simulink model "CiMappedEngine"  (R2021a)
settings: Solver=VariableStepAuto  StartTime=0.0  StopTime=inf  RelTol=1e-3  EnableMultiTasking=on
model workspace (MAT data in the model file):
  AccPwrbp = [0 0]
  AccSpdbp = [300 750]
  Cps = 2
  NCyl = 4
  Pstd = 101325
  Rair = 287.05
  Sinj = 6.45161290323
  TimeCnstECP = 0.125
  TimeCnstEGR = 0.125
  TimeCnstETC = 0.085
  TimeCnstICP = 0.125
  TimeCnstIVL = 0.125
  TimeCnstSWVA = 0.125
  TimeCnstVCR = 0.125
  TimeCnstVGT = 0.15
  TimeCnstVIRL = 0.125
  TimeCnstWGA = 0.15
  Tstd = 293.15
  Vd = 0.0015
  f_air = [0 0 0 0 0 0 0 0 0 0 0 0 ... (320 elements, 20x16)]
  f_air_3d = [0 0 0 0 0 0 0 0 0 0 0 0 ... (960 elements, 20x16x3)]
  f_co = [0 0 0 0 0 0 0 0 0 0 0 0 ... (320 elements, 20x16)]
  f_co2 = [0 0 0 0 0 0 0 0 0 0 0 0 ... (320 elements, 20x16)]
  f_co2_3d = [0 0 0 0 0 0 0 0 0 0 0 0 ... (960 elements, 20x16x3)]
  f_co_3d = [0 0 0 0 0 0 0 0 0 0 0 0 ... (960 elements, 20x16x3)]
  f_eff = [0 0 0 0 0 0 0 0 0 0 0 0 ... (320 elements, 20x16)]
  f_eff_3d = [0 0 0 0 0 0 0 0 0 0 0 0 ... (960 elements, 20x16x3)]
  f_fuel = [0 0 0 0 0 0 0 0 0 0 0 0 ... (320 elements, 20x16)]
  f_fuel_3d = [0 0 0 0 0 0 0 0 0 0 0 0 ... (960 elements, 20x16x3)]
  f_hc = [0 0 0 0 0 0 0 0 0 0 0 0 ... (320 elements, 20x16)]
  f_hc_3d = [0 0 0 0 0 0 0 0 0 0 0 0 ... (960 elements, 20x16x3)]
  f_nox = [0 0 0 0 0 0 0 0 0 0 0 0 ... (320 elements, 20x16)]
  f_nox_3d = [0 0 0 0 0 0 0 0 0 0 0 0 ... (960 elements, 20x16x3)]
  f_pm = [0 0 0 0 0 0 0 0 0 0 0 0 ... (320 elements, 20x16)]
  f_pm_3d = [0 0 0 0 0 0 0 0 0 0 0 0 ... (960 elements, 20x16x3)]
  f_tbrake = [0 15 15 15 15 15 15 15 15 15 15 15 ... (320 elements, 20x16)]
  f_tbrake_3d = [0 4.32139921766 20.7572447114 35.9627269415 49.855265726 62.5657141177 74.4770044016 86.1003984024 97.7334079818 109.479762957 121.326441846 133.101497884 ... (960 elements, 20x16x3)]
  f_tbrake_f_bpt = [0 2.63157894737 5.26315789474 7.89473684211 10.5263157895 13.1578947368 15.7894736842 18.4210526316 21.0526315789 23.6842105263 26.3157894737 28.9473684211 ... (20 elements, 1x20)]
  f_tbrake_n_bpt = [0 1000 1285.71428571 1571.42857143 1857.14285714 2142.85714286 2428.57142857 2714.28571429 3000 3285.71428571 3571.42857143 3857.14285714 ... (16 elements, 1x16)]
  f_tbrake_t_bpt = [0 4.017 21.26 37.37 52.22 65.88 78.77 91.44 104.2 116.8 129.3 141.4 ... (20 elements, 1x20)]
  f_texh = [530.615953519 585.141308787 621.791548793 637.74644696 668.027558986 729.99378178 762.870339995 814.420601609 844.420048857 859.04703204 894.926983859 943.665474082 ... (320 elements, 20x16)]
  f_texh_3d = [358.711368346 410.521929896 465.556483184 518.480956339 566.158596806 618.256764358 675.886138918 720.044246232 742.940029896 751.128194054 760.390444558 779.777710435 ... (960 elements, 20x16x3)]
libraries: autolibpowerinfoutils x1, autolibsharedmappedengines x1
(part 2 of 2)

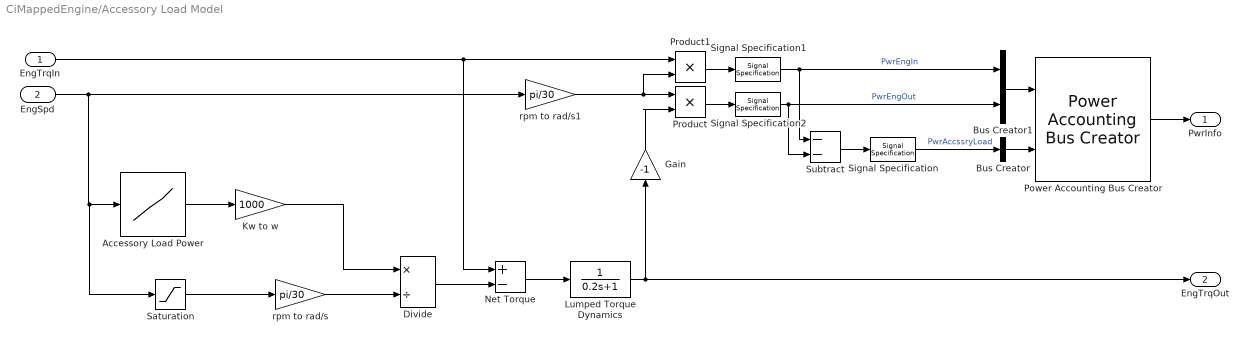
== system CiMappedEngine/Accessory Load Model ==
  EngTrqIn : Inport
  EngSpd : Inport  Port=2
  Accessory Load Power : Lookup_n-D  NumberOfTableDimensions=1  LookupTableObject=''  BreakpointsForDimension1=AccSpdbp  Table=AccPwrbp  ExtrapMethod=Clip  InternalRulePriority=Speed  RndMeth=Simplest  InputSameDT=on
  Bus Creator : BusCreator  Inputs=1
  Bus Creator1 : BusCreator  Inputs=2
  Divide : Product  Inputs=*/
  Gain : Gain  Gain=-1
  Kw to w : Gain  Gain=1000
  Lumped Torque Dynamics : TransferFcn  Denominator=[0.2 1]
  Net Torque : Sum  Inputs=+-
  Power Accounting Bus Creator : autolibpowerinfoutils/Power Accounting Bus Creator  AssctBlkSelPopup=Parent  RefBlkName='libraryname/blkname'  PwrTrnsfrdCheckBox=on  PwrNotTrnsfrdCheckBox=on  PwrStoredCheckBox=off  aMode=aMode
      settings: SourceProductBaseCode=PW,DR,MT,UV,VE
  Product : Product
  Product1 : Product
  Saturation : Saturate  UpperLimit=Inf  LowerLimit=300
  Signal Specification : SignalSpecification  Unit=W
  Signal Specification1 : SignalSpecification  Unit=W
  Signal Specification2 : SignalSpecification  Unit=W
  Subtract : Sum  Inputs=--
  rpm to rad/s : Gain  Gain=pi/30
  rpm to rad/s1 : Gain  Gain=pi/30
  PwrInfo : Outport  VectorParamsAs1DForOutWhenUnconnected=off
  EngTrqOut : Outport  Port=2  Unit=N*m  VectorParamsAs1DForOutWhenUnconnected=off
  wires:
  Divide/1 -> Net Torque/2
  Accessory Load Power/1 -> Kw to w/1
  EngSpd/1 -> Saturation/1, Accessory Load Power/1, rpm to rad/s1/1
  Saturation/1 -> rpm to rad/s/1
  rpm to rad/s/1 -> Divide/2
  Lumped Torque Dynamics/1 -> EngTrqOut/1, Gain/1
  Net Torque/1 -> Lumped Torque Dynamics/1
  Bus Creator/1 -> Power Accounting Bus Creator/2
  Kw to w/1 -> Divide/1
  Bus Creator1/1 -> Power Accounting Bus Creator/1
  EngTrqIn/1 -> Product1/1, Net Torque/1
  Subtract/1 -> Signal Specification/1
  Signal Specification/1 -> Bus Creator/1  "PwrAccssryLoad"
  Power Accounting Bus Creator/1 -> PwrInfo/1
  Product/1 -> Signal Specification2/1
  Product1/1 -> Signal Specification1/1
  rpm to rad/s1/1 -> Product1/2, Product/1
  Signal Specification1/1 -> Subtract/1, Bus Creator1/1  "PwrEngIn"
  Signal Specification2/1 -> Subtract/2, Bus Creator1/2  "PwrEngOut"
  Gain/1 -> Product/2

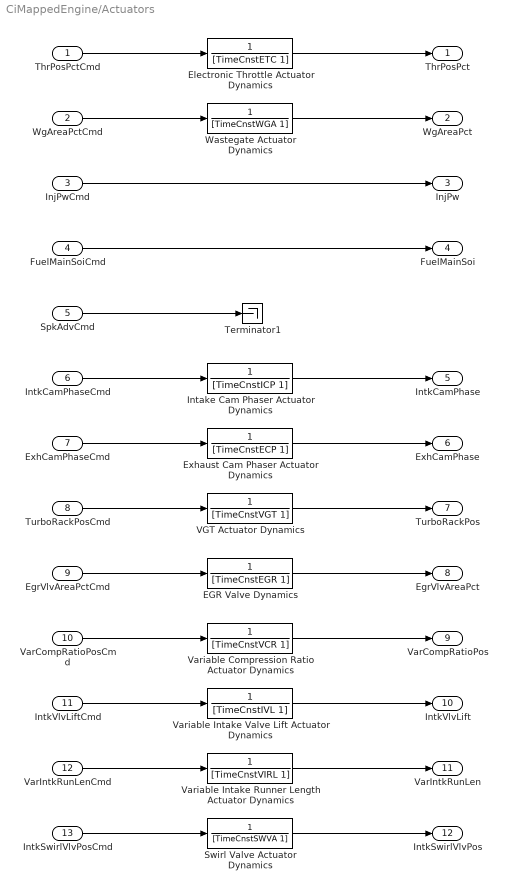
== system CiMappedEngine/Actuators ==
  ThrPosPctCmd : Inport  Unit=%
  WgAreaPctCmd : Inport  Port=2  Unit=%
  InjPwCmd : Inport  Port=3  Unit=ms
  FuelMainSoiCmd : Inport  Port=4  Unit=deg
  SpkAdvCmd : Inport  Port=5  Unit=deg
  IntkCamPhaseCmd : Inport  Port=6  Unit=deg
  ExhCamPhaseCmd : Inport  Port=7  Unit=deg
  TurboRackPosCmd : Inport  Port=8  Unit=1
  EgrVlvAreaPctCmd : Inport  Port=9  Unit=%
  VarCompRatioPosCmd : Inport  Port=10
  IntkVlvLiftCmd : Inport  Port=11
  VarIntkRunLenCmd : Inport  Port=12
  IntkSwirlVlvPosCmd : Inport  Port=13
  EGR Valve Dynamics : TransferFcn  Denominator=[TimeCnstEGR 1]
  Electronic Throttle Actuator Dynamics : TransferFcn  Denominator=[TimeCnstETC 1]
  Exhaust Cam Phaser Actuator Dynamics : TransferFcn  Denominator=[TimeCnstECP 1]
  Intake Cam Phaser Actuator Dynamics : TransferFcn  Denominator=[TimeCnstICP 1]
  Swirl Valve Actuator Dynamics : TransferFcn  Denominator=[TimeCnstSWVA 1]
  Terminator1 : Terminator
  VGT Actuator Dynamics : TransferFcn  Denominator=[TimeCnstVGT 1]
  Variable Compression Ratio Actuator Dynamics : TransferFcn  Denominator=[TimeCnstVCR 1]
  Variable Intake Runner Length Actuator Dynamics : TransferFcn  Denominator=[TimeCnstVIRL 1]
  Variable Intake Valve Lift Actuator Dynamics : TransferFcn  Denominator=[TimeCnstIVL 1]
  Wastegate Actuator Dynamics : TransferFcn  Denominator=[TimeCnstWGA 1]
  ThrPosPct : Outport  Unit=%  VectorParamsAs1DForOutWhenUnconnected=off
  WgAreaPct : Outport  Port=2  Unit=%  VectorParamsAs1DForOutWhenUnconnected=off
  InjPw : Outport  Port=3  VectorParamsAs1DForOutWhenUnconnected=off
  FuelMainSoi : Outport  Port=4  VectorParamsAs1DForOutWhenUnconnected=off
  IntkCamPhase : Outport  Port=5  Unit=deg  VectorParamsAs1DForOutWhenUnconnected=off
  ExhCamPhase : Outport  Port=6  Unit=deg  VectorParamsAs1DForOutWhenUnconnected=off
  TurboRackPos : Outport  Port=7  Unit=1  VectorParamsAs1DForOutWhenUnconnected=off
  EgrVlvAreaPct : Outport  Port=8  Unit=%  VectorParamsAs1DForOutWhenUnconnected=off
  VarCompRatioPos : Outport  Port=9  VectorParamsAs1DForOutWhenUnconnected=off
  IntkVlvLift : Outport  Port=10  VectorParamsAs1DForOutWhenUnconnected=off
  VarIntkRunLen : Outport  Port=11  VectorParamsAs1DForOutWhenUnconnected=off
  IntkSwirlVlvPos : Outport  Port=12  VectorParamsAs1DForOutWhenUnconnected=off
  wires:
  SpkAdvCmd/1 -> Terminator1/1
  EgrVlvAreaPctCmd/1 -> EGR Valve Dynamics/1
  TurboRackPosCmd/1 -> VGT Actuator Dynamics/1
  EGR Valve Dynamics/1 -> EgrVlvAreaPct/1
  VGT Actuator Dynamics/1 -> TurboRackPos/1
  InjPwCmd/1 -> InjPw/1
  VarIntkRunLenCmd/1 -> Variable Intake Runner Length Actuator Dynamics/1
  VarCompRatioPosCmd/1 -> Variable Compression Ratio Actuator Dynamics/1
  IntkCamPhaseCmd/1 -> Intake Cam Phaser Actuator Dynamics/1
  ExhCamPhaseCmd/1 -> Exhaust Cam Phaser Actuator Dynamics/1
  ThrPosPctCmd/1 -> Electronic Throttle Actuator Dynamics/1
  WgAreaPctCmd/1 -> Wastegate Actuator Dynamics/1
  IntkSwirlVlvPosCmd/1 -> Swirl Valve Actuator Dynamics/1
  IntkVlvLiftCmd/1 -> Variable Intake Valve Lift Actuator Dynamics/1
  FuelMainSoiCmd/1 -> FuelMainSoi/1
  Electronic Throttle Actuator Dynamics/1 -> ThrPosPct/1
  Wastegate Actuator Dynamics/1 -> WgAreaPct/1
  Exhaust Cam Phaser Actuator Dynamics/1 -> ExhCamPhase/1
  Intake Cam Phaser Actuator Dynamics/1 -> IntkCamPhase/1
  Swirl Valve Actuator Dynamics/1 -> IntkSwirlVlvPos/1
  Variable Intake Runner Length Actuator Dynamics/1 -> VarIntkRunLen/1
  Variable Intake Valve Lift Actuator Dynamics/1 -> IntkVlvLift/1
  Variable Compression Ratio Actuator Dynamics/1 -> VarCompRatioPos/1
